simulink library "lib_Convection_FalknerSkanTempVary"  (R2015a)
settings: Solver=ode45  StartTime=0.0  StopTime=10.0  RelTol=1e-3
settings Model: Creator=jlkratz  LastModifiedBy=jlkratz

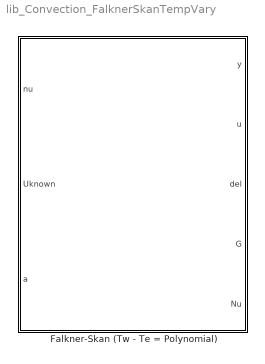
== system lib_Convection_FalknerSkanTempVary ==
  Falkner-Skan (Tw - Te = Polynomial) : Subsystem  mask(TSAT: Falkner-Skan (Tw-Te = Polynomial)){Pr_M=1, beta_M=0, x_Uknown_M=10, x_M=[0.05:0.05:3], n_M=50, imax_M=1000, BN_M=double(gcb)}
      mask prompts: Pr_M "Pr_M - Prandtl number (0.01 < Pr < 40000)"; beta_M "beta_M - Pressure gradient variable (-0.19505 < beta < 1)"; x_Uknown_M "x_Uknown_M - Location of a known velocity along x, Uknown = K*x_Uknown_M^m"; x_M "x_M - Locations along the surface to compute the boundary layer for [mx1]"; n_M "n_M - Number of elements in the boundary layer"; imax_M "imax - Maximum number of iterations of the solver [1x1]"; BN_M "BN_M - Block name"
      mask help:
      | This block implements the Falkner-Skan solution to laminar-boundary-layer flow and addresses temperature variations between the wall and free-stream using the method of indicial solutions (superposition). This block is nearly identical to the "Falkner-Skan (Tw-Te = Constant)" block with the exception of addressing temperature variations. Solution of the hydrodynamic boundary layer is the same. Complexities with the varying wall temperature make it difficult to resolve the temperature profiles within the boundary layer but superposition by indicial solution can be used to estimate the local Nusselt number. Recall that the Falkner-Skan solution generalizes the Blasius solution by allowing U(x) = Kx^m, where K is a m are constants. The pressure gradient (dp/dx) of the flow is expressed using the variable beta.
      |
      | beta = 2*m/(m+1)
      |
      | A positive beta implies a negative or favorable pressure gradient and a negative beta implies a positive or unfavorable pressure gradient. Falkner-Skan flow can be analogous to flow around wedges and corners.
      |
      | -2 <= beta < 0: Flow around an expansion corner of turning angle beta*pi/2
      | beta = -0.19505: onset of separation
      | beta = 0: flat plate
      | 0 < beta <= 2: Flow against a wedge of half-angle beta*pi/2
      | beta = 1: plane stagnation point (180deg wedge)
      |
      | beta's outside this range still have physical meaning which can be used to describe doublet flow and flow toward a point sink. The Falkner-Skan code implemented within the block is capable of handling -0.19505 < beta < 10 but to retain the physical meaning of a flow over a surface which captures separation to stagnation, the beta is restricted to values between -0.19505 to 1.
      |
      | This block solves the laminar flow hydrodynamic boundary layer problem and estimates the local Nusselt number. Resolution of the thermal boundary layer profiles require more attention which often leads to the use of finite-difference methods.
      mask init:
      | %Error/Warning Checking --------------------------------------------------%
      | 
      | %---- Pr_M ----%
      | %Scalar?
      | if isscalar(Pr_M) == 0
      |     Pr_M = 1;
      |     fprintf('Warning in %s: Pr_M must be a scalar. Pr_M has been set equal to 1 for computations.\n',char(BN_M));
      | end
      | %Real?
      | if isreal(Pr_M) == 0
      |     Pr_M = real(Pr_M);
      |     fprintf('Warning in %s: Pr_M must be a real. Pr_M has been set equal to real part of the entered value for computations.\n',char(BN_M));
      | end
      | %Finite?
      | if isfinite(Pr_M) == 0
      |     Pr_M = 1;
      |     fprintf('Warning in %s: Pr_M must be a finite. Pr_M has been set equal to 1 for computations.\n',char(BN_M));
      | end
      | %greater than 0
      | if Pr_M <= 0
      |     Pr_M = 0.01;
      |     fprintf('Warning in %s: Pr_M must be positive. Pr_M has been set equal to 0.01 for computations.\n',char(BN_M));
      | end
      | %Between 0.01 and 40000
      | if Pr_M < 0.01 || Pr_M > 40000
      |     fprintf('Warning in %s: Pr_M is outside of recommended range of Prandtl numbers (0.01 < Pr < 40000). Results could be erroneous.\n',char(BN_M));
      | end
      | %---- beta_M ----%
      | %Scalar?
      | if isscalar(beta_M) == 0
      |     beta_M = 0;
      |     fprintf('Warning in %s: beta_M must be a scalar. beta_M has been set equal to 0 for computations.\n',char(BN_M));
      | end
      | %Real?
      | if isreal(beta_M) == 0
      |     beta_M = real(beta_M);
      |     fprintf('Warning in %s: beta_M must be a real. beta_M has been set equal to real part of the entered value for computations.\n',char(BN_M));
      | end
      | %Finite?
      | if isfinite(beta_M) == 0
      |     beta_M = 0;
      |     fprintf('Warning in %s: beta_M must be a finite. beta_M has been set equal to 0 for computations.\n',char(BN_M));
      | end
      | %greater than -0.19505
      | if beta_M < -0.19505 || beta_M > 1
      |     if beta_M < -0.19505
      |         beta_M = -0.19505;
      |     elseif beta_M > 1
      |         beta_M = 1;
      |     end
      |     fprintf('Warning in %s: beta_M must be between -0.19505 and 1. beta_M has been set equal to the closest value in this range.\n',char(BN_M));
      | end
      | %---- x_Uknown_M ----%
      | %Scalar?
      | if isscalar(x_Uknown_M) == 0
      |     x_Uknown_M = 1;
      |     fprintf('Warning in %s: x_Uknown_M must be a scalar. x_Uknown_M has been set equal to 1 for computations.\n',char(BN_M));
      | end
      | %Real?
      | if isreal(x_Uknown_M) == 0
      |     beta_M = real(x_Uknown_M);
      |     fprintf('Warning in %s: x_Uknown_M must be a real. x_Uknown_M has been set equal to real part of the entered value for computations.\n',char(BN_M));
      | end
      | %Finite?
      | if isfinite(x_Uknown_M) == 0
      |     x_Uknown_M = 1;
      |     fprintf('Warning in %s: x_Uknown_M must be a finite. x_Uknown_M has been set equal to 0 for computations.\n',char(BN_M));
      | end
      | %Positive?
      | if x_Uknown_M <= 0
      |     x_Uknown_M = 1;
      |     fprintf('Warning in %s: x_Uknown_M must be positive and non-zero. x_Uknown_M has been set equal to 1 for computations.\n',char(BN_M));
      | end
      | %---- x_M ----%
      | %Not empty?
      | if isempty(x_M) == 1
      |     x_M = [0.1 0.5 1];
      |     fprintf('Warning in %s: x_M cannot be empty. x_M has been set to [0.1 0.5 1] for computations.\n',char(BN_M));
      | end
      | %1-D array?
      | if min(size(x_M)) ~= 1 || length(size(x_M)) > 2
      |     x_M = [0.1 0.5 1];
      |     fprintf('Warning in %s: x_M must be a 1-D array. x_M has been set to [0.1 0.5 1] for computations.\n',char(BN_M));
      | end
      | %Real?
      | if min(isreal(x_M)) == 0
      |     x_M = real(x_M);
      |     fprintf('Warning in %s: x_M must have all real elements. x_M has been set equal to the real parts of the entered values for computations.\n',char(BN_M));
      | end
      | %Finite?
      | if min(isfinite(x_M)) == 0
      |     x_M = [0.1 0.5 1];
      |     fprintf('Warning in %s: x_M must have all finite elements. x_M has been set equal to [0.1 0.5 1] for computations.\n',char(BN_M));
      | end
      | %Greater than 0?
      | if min(x_M) <= 0
      |     x_M = [0.1 0.5 1];
      |     fprintf('Warning in %s: x_M must have all elements that are greater than 0. x_M has been set equal to [0.1 0.5 1] for computations.\n',char(BN_M));
      | end
      | %Monotonically Increasing?
      | if max(size(x_M)) > 1
      |     if min(diff(x_M)) <= 0
      |         x_M = unique(sort(x_M));
      |         fprintf('Warning in %s: x_M must be a monotonically increasing array. x_M has been put in ascending order with redundant elements removed for computations\n',char(BN_M));
      |     end
      | end
      | %---- n_M ----%
      | %Scalar?
      | if isscalar(n_M) == 0
      |     n_M = 10;
      |     fprintf('Warning in %s: n_M must be a scalar. n_M has been set equal to 10 for computations.\n',char(BN_M));
      | end
      | %Real?
      | if isreal(n_M) == 0
      |     n_M = real(n_M);
      |     fprintf('Warning in %s: n_M must be a real. n_M has been set equal to real part of the entered value for computations.\n',char(BN_M));
      | end
      | %Finite?
      | if isfinite(n_M) == 0
      |     n_M = 10;
      |     fprintf('Warning in %s: n_M must be a finite. n_M has been set equal to 10 for computations.\n',char(BN_M));
      | end
      | %Integer?
      | if rem(n_M,1) > 0
      |     n_M = round(n_M);
      |     fprintf('Warning in %s: n_M must be an integer. n_M has been rounded to the closest integer.\n',char(BN_M));
      | end
      | %Greater than 1?
      | if n_M <= 1
      |     n_M = 2;
      |     fprintf('Warning in %s: n_M must be 2 or greater. n_M has been set equal to 2 for computations.\n',char(BN_M));
      | end
      | %---- imax_M ----%
      | %Scalar?
      | if isscalar(imax_M) == 0
      |     imax_M = 100;
      |     fprintf('Warning in %s: imax_M must be a scalar. imax_M has been set equal to 100 for computations.\n',char(BN_M));
      | end
      | %Real?
      | if isreal(imax_M) == 0
      |     imax_M = real(imax_M);
      |     fprintf('Warning in %s: imax_M must be a real. imax_M has been set equal to real part of the entered value for computations.\n',char(BN_M));
      | end
      | %Finite?
      | if isfinite(imax_M) == 0
      |     imax_M = 100;
      |     fprintf('Warning in %s: imax_M must be a finite. imax_M has been set equal to 100 for computations.\n',char(BN_M));
      | end
      | %Integer?
      | if rem(imax_M,1) > 0
      |     imax_M = round(imax_M);
      |     fprintf('Warning in %s: imax_M must be an integer. imax_M has been rounded to the closest integer.\n',char(BN_M));
      | end
      | %Greater than 0?
      | if imax_M <= 0
      |     imax_M = 100;
      |     fprintf('Warning in %s: imax_M must be 1 or greater. imax_M has been set equal to 100 for computations.\n',char(BN_M));
      | end
      | 
      | %Create eta arrays -------------------------------------------------------%
      | 
      | %Interpolation for etaf (final value in eta)
      | beta_vec = [-0.19505 -0.19 -0.18 -0.15 -0.1 -0.05 0 0.1 0.2 0.3 0.5 0.75 1 1.25 1.5 2 2.5 3 3.5 4 4.5 5 5.5 6 6.5 7 7.5 8 8.5 9 9.5 10];
      | etaf_vec = [8 8 8 8 8 7 7 6.5 6 6 5 5 5 5 5 5 4 3.75 3.5 3 3 3 3 2.5 2.5 2.5 2.5 2.2 2.2 2.1 2.1 2];
      | etaf = interp1(beta_vec,etaf_vec,beta_M,'linear');
      | 
      | %Create eta
      | deta = 0.01;
      | eta_I = [0:deta:etaf];
      | %clearvars -except eta_I beta_M Pr_M
      | 
      | %Interpolation for setting etaf for thermal boundary layer calc
      | BETA_vecT = [-0.19505 0 10];
      | EXP_vecT = [-0.27 -0.33 -0.4];
      | EXP = interp1(BETA_vecT,EXP_vecT,beta_M,'pchip');
      | etaft = etaf*Pr_M^(EXP); %Recommended eta
      | etaft = etaft - rem(etaft,deta);
      | etat_I = [0:deta:etaft];
      | 
      | %Check Warning/Errors
      | %---- eta_I ----%
      | %Not empty?
      | if isempty(eta_I) == 1
      |     fprintf('Warning in %s: eta_I (generated in initialization script) cannot be empty. Re-evaluate parameters.\n',char(BN_M));
      | end
      | %1-D array?
      | if min(size(eta_I)) ~= 1 || length(size(eta_I)) > 2
      |     fprintf('Warning in %s: eta_I (generated in initialization script) must be a 1-D array. Re-evaluate parameters.\n',char(BN_M));
      | end
      | %Real?
      | if min(isreal(eta_I)) == 0
      |     fprintf('Warning in %s: eta_I (generated in initialization script) must have all real elements. Re-evaluate parameters.\n',char(BN_M));
      | end
      | %Finite?
      | if min(isfinite(eta_I)) == 0
      |     fprintf('Warning in %s: eta_I (generated in initialization script) must have all finite elements. Re-evaluate parameters.\n',char(BN_M));
      | end
      | %Greater than 0?
      | if min(eta_I) < 0
      |     fprintf('Warning in %s: eta_I (generated in initialization script) must have all elements that are greater than 0. Re-evaluate parameters.\n',char(BN_M));
      | end
      | %Monotonically Increasing?
      | if max(size(eta_I)) > 1
      |     if min(diff(eta_I)) <= 0
      |         fprintf('Warning in %s: eta_I (generated in initialization script) must be a monotonically increasing array. Re-evaluate parameters.\n',char(BN_M));
      |     end
      | end
      | %---- etat_I ----%
      | %Not empty?
      | if isempty(etat_I) == 1
      |     fprintf('Warning in %s: eta_I (generated in initialization script) cannot be empty. Re-evaluate parameters.\n',char(BN_M));
      | end
      | %1-D array?
      | if min(size(etat_I)) ~= 1 || length(size(etat_I)) > 2
      |     fprintf('Warning in %s: etat_I (generated in initialization script) must be a 1-D array. Re-evaluate parameters.\n',char(BN_M));
      | end
      | %Real?
      | if min(isreal(etat_I)) == 0
      |     fprintf('Warning in %s: etat_I (generated in initialization script) must have all real elements. Re-evaluate parameters.\n',char(BN_M));
      | end
      | %Finite?
      | if min(isfinite(etat_I)) == 0
      |     fprintf('Warning in %s: etat_I (generated in initialization script) must have all finite elements. Re-evaluate parameters.\n',char(BN_M));
      | end
      | %Greater than 0?
      | if min(etat_I) < 0
      |     fprintf('Warning in %s: etat_I (generated in initialization script) must have all elements that are greater than 0. Re-evaluate parameters.\n',char(BN_M));
      | end
      | %Monotonically Increasing?
      | if max(size(etat_I)) > 1
      |     if min(diff(etat_I)) <= 0
      |         fprintf('Warning in %s: etat_I (generated in initialization script) must be a monotonically increasing array. Re-evaluate parameters.\n',char(BN_M));
      |     end
      | end
      mask Help: web(which('Convection_TSAT_FalknerSkanTempVary.html'),'-helpbrowser')

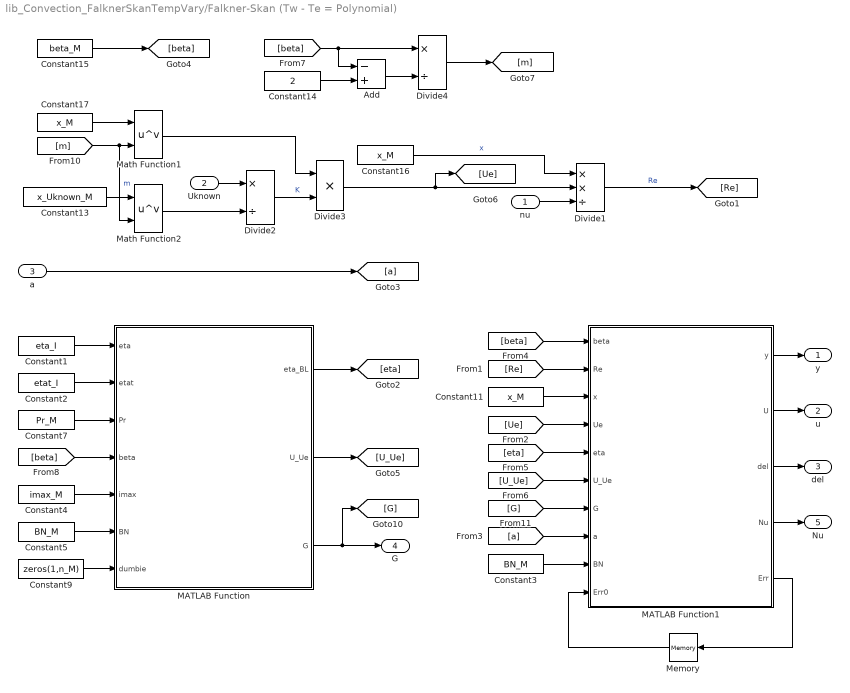
== system lib_Convection_FalknerSkanTempVary/Falkner-Skan (Tw - Te = Polynomial) ==
  nu : Inport
  Uknown : Inport  Port=2
  a : Inport  Port=3
  Add : Sum  Inputs=-+
  Constant1 : Constant  Value=eta_I
  Constant11 : Constant  Value=x_M
  Constant13 : Constant  Value=x_Uknown_M
  Constant14 : Constant  Value=2
  Constant15 : Constant  Value=beta_M
  Constant16 : Constant  Value=x_M
  Constant17 : Constant  Value=x_M
  Constant2 : Constant  Value=etat_I
  Constant3 : Constant  Value=BN_M
  Constant4 : Constant  Value=imax_M
  Constant5 : Constant  Value=BN_M
  Constant7 : Constant  Value=Pr_M
  Constant9 : Constant  Value=zeros(1,n_M)
  Divide1 : Product  Inputs=**/
  Divide2 : Product  Inputs=*/
  Divide3 : Product  Inputs=**
  Divide4 : Product  Inputs=*/
  MATLAB Function : MATLAB Function  TreatAsAtomicUnit=on
  MATLAB Function1 : MATLAB Function  TreatAsAtomicUnit=on
  Math Function1 : Math  Operator=pow  SaturateOnIntegerOverflow=on
  Math Function2 : Math  Operator=pow  SaturateOnIntegerOverflow=on
  Memory : Memory  X0=zeros(1,14)
  y : Outport
  u : Outport  Port=2
  del : Outport  Port=3
  G : Outport  Port=4
  Nu : Outport  Port=5
  wires:
  [G] -> MATLAB Function1/7(G)
  [U_Ue] -> MATLAB Function1/6(U_Ue)
  [eta] -> MATLAB Function1/5(eta)
  [a] -> MATLAB Function1/8(a)
  [Ue] -> MATLAB Function1/4(Ue)
  Constant11/1 -> MATLAB Function1/3(x)
  [Re] -> MATLAB Function1/2(Re)
  MATLAB Function1/3(del) -> del/1
  MATLAB Function1/4(Nu) -> Nu/1
  MATLAB Function1/1(y) -> y/1
  MATLAB Function1/2(U) -> u/1
  [beta] -> MATLAB Function1/1(beta)
  Constant9/1 -> MATLAB Function/7(dumbie)
  MATLAB Function/2(U_Ue) -> [U_Ue]
  MATLAB Function/1(eta_BL) -> [eta]
  a/1 -> [a]
  Constant7/1 -> MATLAB Function/3(Pr)
  [beta] -> MATLAB Function/4(beta)
  Constant2/1 -> MATLAB Function/2(etat)
  MATLAB Function/3(G) -> G/1, [G]
  Constant5/1 -> MATLAB Function/6(BN)
  Constant4/1 -> MATLAB Function/5(imax)
  Constant1/1 -> MATLAB Function/1(eta)
  Divide3/1 -> Divide1/2, [Ue]
  [m] -> Math Function2/2, Math Function1/2  "m"
  Constant17/1 -> Math Function1/1
  nu/1 -> Divide1/3
  Constant16/1 -> Divide1/1  "x"
  Divide1/1 -> [Re]  "Re"
  Uknown/1 -> Divide2/1
  Divide2/1 -> Divide3/2  "K"
  Math Function1/1 -> Divide3/1
  [beta] -> Add/1, Divide4/1
  Constant14/1 -> Add/2
  Add/1 -> Divide4/2
  Divide4/1 -> [m]
  Constant15/1 -> [beta]
  Constant13/1 -> Math Function2/1
  Math Function2/1 -> Divide2/2
  MATLAB Function1/5(Err) -> Memory/1
  Memory/1 -> MATLAB Function1/10(Err0)
  Constant3/1 -> MATLAB Function1/9(BN)

== matlab function lib_Convection_FalknerSkanTempVary/Falkner-Skan (Tw - Te = Polynomial)/MATLAB Function1 ==
  data: beta input; y output; Re input; x input; Ue input; eta input; U_Ue input; G input; a input; BN input; U output; del output; Nu output; Err0 input; Err output
function [y, U, del, Nu, Err] = BoundaryLayerCalcs(beta, Re, x, Ue, eta, U_Ue, G, a, BN, Err0)
%#codegen

%Description
% This function block computes dimensional quantities and forms the outputs

%Inputs:
% beta - pressure gradient variable [1x1]
% Re - Reynolds number [mx1]
% x - spatial variable along the surface [mx1]
% Ue - free-stream velocity [mx1]
% G - Falkner-Skan Heat Transfer parameter [nx1]
% a - array with polynomial coefficients for Tw-Te [px1]

%Outputs:
% y - dimensional y-coordinates for the velocity profile [nxm]
% U - velocity profile U(x,y) [nxm]
% del - hydrodynamic boundary layer thickness, del(x) [mx1]
% Nu - Nusselt number, Nu(x)[mx1]

%Error/Warning Checks ----------------------------------------------------%

Err = Err0;
ErrNum = 1;
%---- Re ----%
%Not empty?
if isempty(Re) == 1 &&  Err(ErrNum) == 0
    Err(ErrNum) = 1;
    fprintf('Warning in %s: Re is an empty array. It is suggested you check nu, Uknown, x_M, and x_Uknown_M for sources of the error.\n',char(BN));
end
ErrNum = ErrNum + 1;
%1D array the length of x?
if (min(size(Re)) > 1 || length(size(Re)) > 2) && Err(ErrNum) == 0
    Err(ErrNum) = 1;
    fprintf('Warning in %s: Re must be a 1-D array. It is suggested you check nu, Uknown, x_M, and x_Uknown_M for sources of the error.\n',char(BN));
end
ErrNum = ErrNum + 1;
%Real?
if min(isreal(Re)) < 1 && Err(ErrNum) == 0
    Err(ErrNum) = 1;
    fprintf('Warning in %s: Re must have all real elements. It is suggested you check nu, Uknown, x_M, and x_Uknown_M for sources of the error.\n',char(BN));
end
ErrNum = ErrNum + 1;
%Finite?
if min(isfinite(Re)) < 1 && Err(ErrNum) == 0
    Err(ErrNum) = 1;
    fprintf('Warning in %s: Re must have all finite elements. It is suggested you check nu, Uknown, x_M, and x_Uknown_M for sources of the error.\n',char(BN));
end
ErrNum = ErrNum + 1;
%Positive?
if min(Re) <= 0 && Err(ErrNum) == 0
    Err(ErrNum) = 1;
    fprintf('Warning in %s: Re must be greater than 0. It is suggested you check nu, Uknown, x_M, and x_Uknown_M for sources of the error.\n',char(BN));
end
ErrNum = ErrNum + 1;
%---- Ue ----%
%Not empty?
if isempty(Ue) == 1 &&  Err(ErrNum) == 0
    Err(ErrNum) = 1;
    fprintf('Warning in %s: Ue is an empty array. It is suggested you check Uknown and x_Uknown_M for sources of the error.\n',char(BN));
end
ErrNum = ErrNum + 1;
%1D array the length of x?
if (min(size(Ue)) > 1 || length(size(Ue)) > 2) && Err(ErrNum) == 0
    Err(ErrNum) = 1;
    fprintf('Warning in %s: Ue must be a 1-D array. It is suggested you check Uknown and x_Uknown_M for sources of the error.\n',char(BN));
end
ErrNum = ErrNum + 1;
%Real?
if min(isreal(Ue)) < 1 && Err(ErrNum) == 0
    Err(ErrNum) = 1;
    fprintf('Warning in %s: Ue must have all real elements. It is suggested you check Uknown and x_Uknown_M for sources of the error.\n',char(BN));
end
ErrNum = ErrNum + 1;
%Finite?
if min(isfinite(Ue)) < 1 && Err(ErrNum) == 0
    Err(ErrNum) = 1;
    fprintf('Warning in %s: Ue must have all finite elements. It is suggested you check Uknown and x_Uknown_M for sources of the error.\n',char(BN));
end
ErrNum = ErrNum + 1;
%Positive?
if min(Ue) <= 0 && Err(ErrNum) == 0
    Err(ErrNum) = 1;
    fprintf('Warning in %s: Ue must be greater than 0. It is suggested you check Uknown and x_Uknown_M for sources of the error.\n',char(BN));
end
ErrNum = ErrNum + 1;
%---- a ----%
%Not empty?
if isempty(a) == 1 && Err(ErrNum) == 0
    Err(ErrNum) = 1;
    fprintf('Warning in %s: a is empty.\n',char(BN));
end
ErrNum = ErrNum + 1;
%1D array > 1 element
if (length(size(a)) > 2 || min(size(a)) ~= 1) && length(a) < 2 && Err(ErrNum) == 0
    Err(ErrNum) = 1;
    fprintf('Warning in %s: a must be a 1D array with at least 2 elements.\n',char(BN));
end
ErrNum = ErrNum + 1;
%Real?
if min(isreal(a)) < 1 && Err(ErrNum) == 0
    Err(ErrNum) = 1;
    fprintf('Warning in %s: a must have all real elements.\n',char(BN));
end
ErrNum = ErrNum + 1;
%Finite?
if min(isfinite(a)) < 1 && Err(ErrNum) == 0
    Err(ErrNum) = 1;
    fprintf('Warning in %s: a must have all finitie elements.\n',char(BN));
end

%Initialize Outputs ------------------------------------------------------%

y = zeros(length(eta),length(x));
U = zeros(length(eta),length(x));
del = zeros(1,length(x));
Nu = zeros(1,length(x));

%Calculations ------------------------------------------------------------%

m = beta/(2 - beta);
for i = 1:length(eta)
    for j = 1:length(x)
        y(i,j) = eta(i)*x(j)/sqrt((m+1)/2*Re(j));
        U(i,j) = U_Ue(i)*Ue(j);
    end
end
for j = 1:length(x)
    del(j) = y(end,j);
end

qwx_k = zeros(1,length(x));
for j = 1:length(x)
    SUM = 0;
    for i = 2:length(a)
        SUM = SUM + (4/3)*(i-1)*a(i)*x(j)^(i-1)*(gamma(4*(i-1)/3)*gamma(2/3)/(gamma(4*(i-1)/3 + 2/3)));
    end
    qwx_k(j) = sqrt((m+1)/2)*G*Re(j)^(1/2)*(a(1) + SUM);
    TwmTe = 0;
    for i = 1:length(a)
        TwmTe = TwmTe + a(i)*x(j)^(i-1);
    end
    Nu(j) = qwx_k(j)/(TwmTe);
end

== matlab function lib_Convection_FalknerSkanTempVary/Falkner-Skan (Tw - Te = Polynomial)/MATLAB Function ==
  data: eta input; etat input; eta_BL output; Pr input; beta input; U_Ue output; imax input; BN input; G output; dumbie input
function [eta_BL, U_Ue, G] = FalknerSkan( eta, etat, Pr, beta, imax, BN, dumbie )
%#codegen

%Inputs
% eta - 
% etat - 
% x - Location from leading edge/start of boundary layer (BL) [mx1]
% Re - Reynolds number [1x1]
% Pr - Prandtl number [1x1]
% beta - Pressure gradient parameter [1x1]
% imax - Maximum number of iterations before solver gives up [1x1]
% BN - Block name

%Outputs
% y - Spatial array in perpendicular direction to the surface - corresponds
%   to U_Ue [nx1]
% U_Ue - Array of local velocity over the free stream or edge velocity 
%   [nx1]
% del - Boundary layer thickness [1x1]
% yt - Spatial array in perpendicular direction to the surface - 
%   corresponds to TmTe_TwmTe [nx1]
% TmTe_TwmTe - Array of (T - Te)/(Tw - Te) where T is the local
%   temperature, Te is the edge temperature, and Tw is the wall temperature
%   [nx1]
% delt - Thermal boundary layer thickness [1x1]

%Variable Definitions ----------------------------------------------------%

%Interpolation arrays for initializing f''(0) in Falkner-Skan Solution
beta_vec = [-0.19505 -0.19 -0.18 -0.15 -0.1 -0.05 0 0.1 0.2 0.3 0.5 0.75 1 1.25 1.5 2 2.5 3 3.5 4 4.5 5 5.5 6 6.5 7 7.5 8 8.5 9 9.5 10];
d2fdeta2_vec = [0 0.067243391282662 0.119 0.215415686186556 0.324359798859230 0.408681194861991 0.48015 0.600910783774823 0.702648045200580 0.79212 0.947023988563495 1.111322201972795 1.25449 1.382949557507723 1.500421070700432 1.711211 1.898566593995162 2.06887312 2.226063730827834 2.372761821 2.510817977693458 2.64159848175 2.766141390500639 2.885262457451 2.999610507546221 3.109718661201 3.216023381125941 3.31889471170345 3.418643437891173 3.51553898188481 3.609811791013788 3.701663533812665];
              
%Falkner-Skan Solution ---------------------------------------------------%

%Initial Conditions
x0 = interp1(beta_vec,d2fdeta2_vec,beta,'pchip'); %f''(0)
y0 = 0; %f'(0) = 0; <-- U/Ue
z0 = 0; %f(0) = 0; <-- Stream Function

%Initialize Solution Arrays
f = [z0, zeros(1,length(eta)-1)]; %f(eta) = stream function
dfdeta = [y0, zeros(1,length(eta)-1)]; %f'(eta) = U/Ue
d2fdeta2 = [x0, zeros(1,length(eta)-1)]; %f''(eta)

%Iterative Solution Until U/Ue at edge --> 1, and f'' at edge --> 0
X1 = x0 - 0.2;
X2 = x0 + 0.2;
cnt = 0;
exitCond = 0;
while exitCond < 0.5
    %fprintf('U cnt: %-1.0f\n',cnt)
    h = eta(2)-eta(1);
    x = [x0, zeros(1,length(eta)-1)];
    y = [y0, zeros(1,length(eta)-1)];
    z = [z0, zeros(1,length(eta)-1)];
    for i = 1:length(eta)-1
        k1x = -z(i)*x(i) - beta*(1 - y(i)^2);
        k1y = x(i);
        k1z = y(i);
        k2x = -(z(i)+.5*k1z*h)*(x(i)+.5*k1x*h) - beta*(1 - (y(i)+.5*k1y*h)^2);
        k2y = x(i)+.5*k1x*h;
        k2z = y(i)+.5*k1y*h;
        k3x = -(z(i)+.5*k2z*h)*(x(i)+.5*k2x*h) - beta*(1 - (y(i)+.5*k2y*h)^2);
        k3y = x(i)+.5*k2x*h;
        k3z = y(i)+.5*k2y*h;
        k4x = -(z(i)+k3z*h)*(x(i)+k3x*h) - beta*(1 - (y(i)+k3y*h)^2);
        k4y = x(i)+k3x*h;
        k4z = y(i)+k3y*h;
        x(i+1) = x(i)+(1/6)*(k1x+2*k2x+2*k3x+k4x)*h;
        y(i+1) = y(i)+(1/6)*(k1y+2*k2y+2*k3y+k4y)*h;
        z(i+1) = z(i)+(1/6)*(k1z+2*k2z+2*k3z+k4z)*h;
        d2fdeta2(i+1) = x(i+1);
        dfdeta(i+1) = y(i+1);
        f(i+1) = z(i+1);
    end
    if abs(1 - dfdeta(end)) > 0.0001 || abs(d2fdeta2(end)) > 0.001
        if dfdeta(end) < 1
            X1 = x0;
        else
            X2 = x0;
        end
        x0 = (X1 + X2)/2;
        cnt = cnt + 1;
        if cnt >= imax
            exitCond = 1;
        end
    else
        exitCond = 1;
    end
end

%Boundary Layer Calculation
eta_e = 99; %initialize
for i = 1:length(eta)-1
    if dfdeta(i) < 0.99 && dfdeta(i+1) >= 0.99
        %eta at which U/Ue = 0.99
        eta_e = (0.99 - dfdeta(i))/(dfdeta(i+1) - dfdeta(i)) * (eta(i+1) - eta(i)) + eta(i);
    end
end

%Create boundary layer arrays
eta_BL = zeros(1,length(dumbie));
U_Ue = zeros(1,length(dumbie));
deta = eta_e/(length(dumbie)-1);
eta_BL(1) = 0;
for i = 2:length(dumbie)
    eta_BL(i) = eta_BL(i-1) + deta;
    U_Ue(i) = interp1(eta,dfdeta,eta_BL(i),'linear'); %U/Ue
end

%Thermal Falkner-Skan Solution -------------------------------------------%

%Extend/Truncate f to match etat
ft = zeros(1,length(etat));
for i = 1:length(etat)
    if etat(i) < eta(end)
        ft(i) = f(i);
    else
        slope = (f(end) - f(end-1))/(eta(end) - eta(end-1));
        ft(i) = f(end) + slope*(etat(i) - eta(end));
    end
end

%Initial Conditions
etat_int = linspace(0,etat(end),100);
ft_int = interp1(etat,ft,etat_int,'linear');
INT = [0, zeros(1,length(etat_int)-1)];
for i = 2:length(etat_int)
    INT(i) = trapz(etat_int(1:i),ft_int(1:i));
end
G = 1/trapz(etat_int,exp(-Pr*INT));
